simulink library "Multi Model Toolbox"  (R2024a)
settings: Solver=VariableStepAuto  StartTime=0.0  StopTime=10.0  RelTol=1e-3
settings Model: Creator=jdazo054  LastModifiedBy=jdazo054

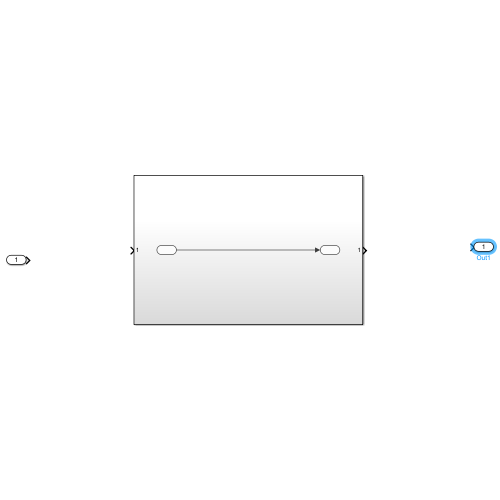
[thumbnail: Simulink's stored preview of the top-level diagram]
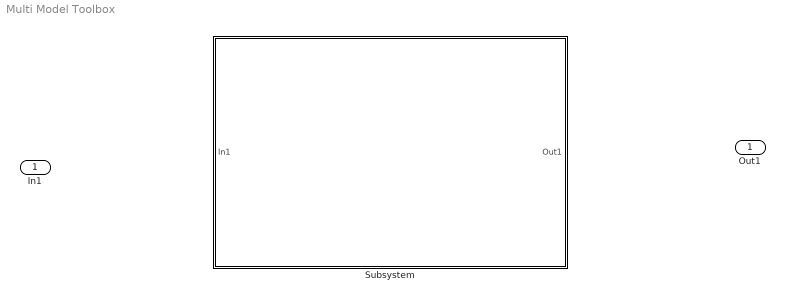
== system Multi Model Toolbox ==
  In1 : Inport
  Subsystem : Subsystem
  Out1 : Outport

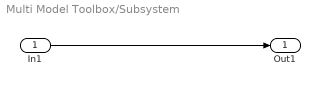
== system Multi Model Toolbox/Subsystem ==
  In1 : Inport
  Out1 : Outport
  wires:
  In1/1 -> Out1/1
